simulink model "test_model_new1"  (R2018a)
settings: Solver=VariableStepAuto  StartTime=0.0  StopTime=7.1  RelTol=1e-3
values from neighbouring files (symbols this model uses):
  A = sys_d.A    [discreteTest.m]    (also in discreteTestAttacked.m)
  B = sys_d.B    [discreteTest.m]    (also in discreteTestAttacked.m)
  C = sys_d.C    [discreteTest.m]    (also in discreteTestAttacked.m)
  K = [   5.261, -0.023 ... (first row only)    [discreteTest.m]    (also in discreteTestAttacked.m)
  steeringAngle = zeros(1, time)    [discreteTest.m]    (also in discreteTestAttacked.m)
  Ts = 0.04    [discreteTest.m]    (also in discreteTestAttacked.m)
undefined symbols (not defined in the file or in its folder): canChannel, L
libraries: canlib x10, canmsglib x8, simulink x6
settings Model: Creator=Shreyash  LastModifiedBy=Shreyash

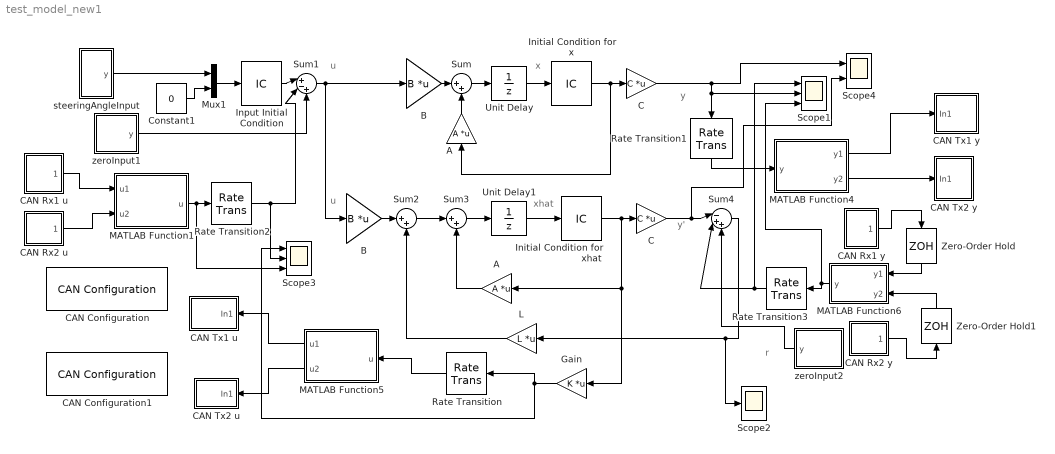
== system test_model_new1 ==
  note: y
  note: r
  note: y'
  note: u
  note: u
  note: x
  note: xhat
  A : Gain  Gain=A  Multiplication=Matrix(K*u)
  "A " : Gain  Gain=A  Multiplication=Matrix(K*u)
  B : Gain  Gain=B  Multiplication=Matrix(K*u)
  "B " : Gain  Gain=B  Multiplication=Matrix(K*u)
  C : Gain  Gain=C  Multiplication=Matrix(K*u)
  "C " : Gain  Gain=C  Multiplication=Matrix(K*u)
  CAN Configuration : canlib/CAN Configuration  BlockHandle=1047.0007  DeviceMenu=MathWorks Virtual 1 (Channel 1)  Device=MathWorks Virtual 1 (Channel 1)  ObjConstructor=canChannel('MathWorks', 'Virtual 1', 1)  BusSpeed=500000  EnableBitParameters=off  AckMode=Normal
      settings: SourceProductBaseCode=VN
  CAN Configuration1 : canlib/CAN Configuration  BlockHandle=1049.0009  DeviceMenu=MathWorks Virtual 1 (Channel 2)  Device=MathWorks Virtual 1 (Channel 2)  ObjConstructor=canChannel('MathWorks', 'Virtual 1', 2)  BusSpeed=500000  EnableBitParameters=off  AckMode=Normal
      settings: SourceProductBaseCode=VN
  CAN Rx1 u : Subsystem
  CAN Rx1 y : Subsystem
  CAN Rx2 u : Subsystem
  CAN Rx2 y : Subsystem
  CAN Tx1 u : Subsystem
  CAN Tx1 y : Subsystem
  CAN Tx2 u : Subsystem
  CAN Tx2 y : Subsystem
  Constant1 : Constant  Value=0
  Gain : Gain  Gain=K  Multiplication=Matrix(K*u)
  Initial Condition for x : InitialCondition  Value=[0;0]
  Initial Condition for xhat : InitialCondition  Value=[0;0]
  Input Initial Condition : InitialCondition  Value=[0;0]
  L : Gain  Gain=L  Multiplication=Matrix(K*u)
  MATLAB Function1 : MATLAB Function  TreatAsAtomicUnit=on
  MATLAB Function4 : MATLAB Function  TreatAsAtomicUnit=on
  MATLAB Function5 : MATLAB Function  TreatAsAtomicUnit=on
  MATLAB Function6 : MATLAB Function  TreatAsAtomicUnit=on
  Mux1 : Mux  Inputs=2
  Rate Transition : RateTransition  Deterministic=off  InitialCondition=Ts/500  OutPortSampleTime=Ts/500
  Rate Transition1 : RateTransition  Deterministic=off  InitialCondition=Ts  OutPortSampleTime=Ts
  Rate Transition2 : RateTransition  Deterministic=off  InitialCondition=0.0004  OutPortSampleTime=Ts
  Rate Transition3 : RateTransition  Deterministic=off  InitialCondition=0.0004  OutPortSampleTime=Ts/2
  Scope1 : Scope  NumInputPorts=3
  Scope2 : Scope
  Scope3 : Scope  NumInputPorts=3
  Scope4 : Scope  NumInputPorts=2
  Sum : Sum  Inputs=|++
  Sum1 : Sum  Inputs=|+-+
  Sum2 : Sum  Inputs=|++
  Sum3 : Sum  Inputs=|++
  Sum4 : Sum  Inputs=|-++
  Unit Delay : UnitDelay  SampleTime=-1
  Unit Delay1 : UnitDelay  SampleTime=-1
  Zero-Order Hold : ZeroOrderHold  SampleTime=Ts/100
  Zero-Order Hold1 : ZeroOrderHold  SampleTime=Ts/100
  steeringAngleInput : Subsystem
  zeroInput1 : Subsystem
  zeroInput2 : Subsystem
  wires:
  "B "/1 -> Sum/1
  Unit Delay/1 -> Initial Condition for x/1
  Sum/1 -> Unit Delay/1
  "A "/1 -> Sum/2
  Constant1/1 -> Mux1/2
  B/1 -> Sum2/1
  Sum2/1 -> Sum3/1
  Sum3/1 -> Unit Delay1/1
  Unit Delay1/1 -> Initial Condition for xhat/1
  L/1 -> Sum2/2
  A/1 -> Sum3/2
  Initial Condition for x/1 -> "C "/1, "A "/1
  C/1 -> Scope4/2, Sum4/1
  Initial Condition for xhat/1 -> C/1, A/1, Gain/1
  Mux1/1 -> Input Initial Condition/1
  Input Initial Condition/1 -> Sum1/1
  Gain/1 -> Scope3/1, Rate Transition/1
  Rate Transition/1 -> MATLAB Function5/1(u)
  "C "/1 -> Rate Transition1/1, Scope1/2, Scope4/1
  MATLAB Function5/1(u1) -> CAN Tx1 u/1(In1)
  MATLAB Function5/2(u2) -> CAN Tx2 u/1(In1)
  steeringAngleInput/1(y) -> Mux1/1
  zeroInput1/1(y) -> Sum1/3
  zeroInput2/1(y) -> Sum4/3
  CAN Rx2 u/1(Data) -> MATLAB Function1/2(u2)
  CAN Rx1 u/1(Data) -> MATLAB Function1/1(u1)
  MATLAB Function1/1(u) -> Scope3/3, Rate Transition2/1
  Sum1/1 -> "B "/1, B/1
  Sum4/1 -> Scope2/1, L/1
  Rate Transition2/1 -> Sum1/2, Scope3/2
  MATLAB Function6/1(y) -> Rate Transition3/1, Scope1/3
  Rate Transition3/1 -> Scope1/1, Sum4/2
  MATLAB Function4/1(y1) -> CAN Tx1 y/1(In1)
  MATLAB Function4/2(y2) -> CAN Tx2 y/1(In1)
  CAN Rx1 y/1(Data) -> Zero-Order Hold/1
  Zero-Order Hold/1 -> MATLAB Function6/1(y1)
  CAN Rx2 y/1(Data) -> Zero-Order Hold1/1
  Zero-Order Hold1/1 -> MATLAB Function6/2(y2)
  Rate Transition1/1 -> MATLAB Function4/1(y)

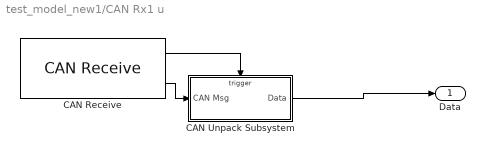
== system test_model_new1/CAN Rx1 u ==
  CAN Receive : canlib/CAN Receive  BlockHandle=1067.0006  DeviceMenu=MathWorks Virtual 1 (Channel 2)  Device=MathWorks Virtual 1 (Channel 2)  ObjConstructor=canChannel('MathWorks', 'Virtual 1', 2)  EnableStandardIDsFilter=off  StandardIDs=201  EnableExtendedIDsFilter=off  ExtendedIDs=0  SampleTime=0.0004  MsgsPerTimestep=all  StdIDsCombo=Allow only  ExtIDsCombo=Block all  InternalFilterUpdateStatus=on  BusOutput=off
      settings: SourceProductBaseCode=VN
  CAN Unpack Subsystem : Subsystem  TreatAsAtomicUnit=on
  Data : Outport  VectorParamsAs1DForOutWhenUnconnected=on
  wires:
  CAN Receive/2 -> CAN Unpack Subsystem/1(CAN Msg)
  CAN Receive/1 -> CAN Unpack Subsystem/Trigger
  CAN Unpack Subsystem/1(Data) -> Data/1

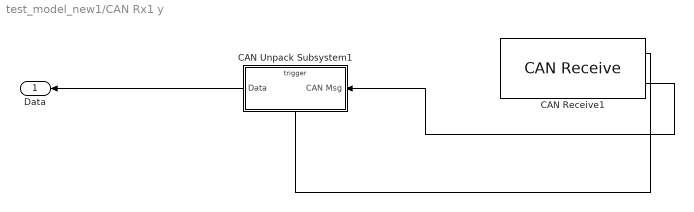
== system test_model_new1/CAN Rx1 y ==
  CAN Receive1 : canlib/CAN Receive  BlockHandle=1080.0006  DeviceMenu=MathWorks Virtual 1 (Channel 2)  Device=MathWorks Virtual 1 (Channel 2)  ObjConstructor=canChannel('MathWorks', 'Virtual 1', 2)  EnableStandardIDsFilter=off  StandardIDs=100  EnableExtendedIDsFilter=off  ExtendedIDs=0  SampleTime=0.0004  MsgsPerTimestep=all  StdIDsCombo=Allow only  ExtIDsCombo=Block all  InternalFilterUpdateStatus=on  BusOutput=off
      settings: SourceProductBaseCode=VN
  CAN Unpack Subsystem1 : Subsystem  TreatAsAtomicUnit=on
  Data : Outport  SampleTime=Ts  VectorParamsAs1DForOutWhenUnconnected=on
  wires:
  CAN Receive1/1 -> CAN Unpack Subsystem1/Trigger
  CAN Receive1/2 -> CAN Unpack Subsystem1/1(CAN Msg)
  CAN Unpack Subsystem1/1(Data) -> Data/1

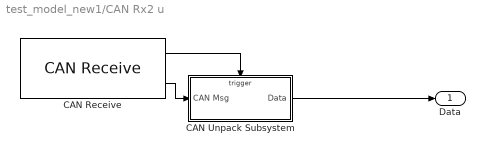
== system test_model_new1/CAN Rx2 u ==
  CAN Receive : canlib/CAN Receive  BlockHandle=1093.0005  DeviceMenu=MathWorks Virtual 1 (Channel 2)  Device=MathWorks Virtual 1 (Channel 2)  ObjConstructor=canChannel('MathWorks', 'Virtual 1', 2)  EnableStandardIDsFilter=off  StandardIDs=202  EnableExtendedIDsFilter=off  ExtendedIDs=0  SampleTime=0.0004  MsgsPerTimestep=all  StdIDsCombo=Allow only  ExtIDsCombo=Block all  InternalFilterUpdateStatus=on  BusOutput=off
      settings: SourceProductBaseCode=VN
  CAN Unpack Subsystem : Subsystem  TreatAsAtomicUnit=on
  Data : Outport  VectorParamsAs1DForOutWhenUnconnected=on
  wires:
  CAN Receive/2 -> CAN Unpack Subsystem/1(CAN Msg)
  CAN Receive/1 -> CAN Unpack Subsystem/Trigger
  CAN Unpack Subsystem/1(Data) -> Data/1

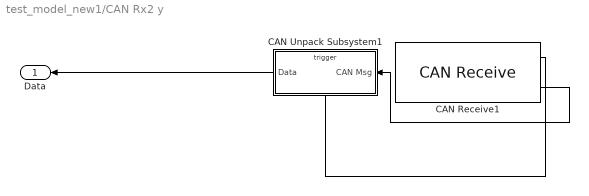
== system test_model_new1/CAN Rx2 y ==
  CAN Receive1 : canlib/CAN Receive  BlockHandle=1201.0005  DeviceMenu=MathWorks Virtual 1 (Channel 2)  Device=MathWorks Virtual 1 (Channel 2)  ObjConstructor=canChannel('MathWorks', 'Virtual 1', 2)  EnableStandardIDsFilter=off  StandardIDs=101  EnableExtendedIDsFilter=off  ExtendedIDs=0  SampleTime=0.0004  MsgsPerTimestep=all  StdIDsCombo=Allow only  ExtIDsCombo=Block all  InternalFilterUpdateStatus=on  BusOutput=off
      settings: SourceProductBaseCode=VN
  CAN Unpack Subsystem1 : Subsystem  TreatAsAtomicUnit=on
  Data : Outport  SampleTime=Ts  VectorParamsAs1DForOutWhenUnconnected=on
  wires:
  CAN Receive1/1 -> CAN Unpack Subsystem1/Trigger
  CAN Receive1/2 -> CAN Unpack Subsystem1/1(CAN Msg)
  CAN Unpack Subsystem1/1(Data) -> Data/1

== system test_model_new1/CAN Tx1 u ==
  In1 : Inport
  CAN Pack : canmsglib/CAN Pack  MsgList=(none)  MsgName=CAN Msg  MsgIDType=Standard (11-bit identifier)  MsgIdentifier=201  MsgLength=8  SignalInfo=signal$0$64$1$4$1$0$1$0$-Inf$Inf$#  NSignals=1  StartBits=str2num('[int32(0)]')  SignalSizes=str2num('[int32(64)]')  ByteOrders=str2num('[int32(1)]')  DataTypes=str2num('[int32(4)]')  MultiplexTypes=str2num('[int32(1)]')  MultiplexValues=str2num('[double(0)]')  Factors=str2num('[double(1)]')  Offsets=str2num('[double(0)]')  Minimums=str2num('[double(-Inf)]')  Maximums=str2num('[double(Inf)]')  Remote=off  ApplyMinMax=off  BusOutput=off
      settings: SourceProductBaseCode=ME,VN  DataFormat=manually specified signals
  CAN Transmit : canlib/CAN Transmit  BlockHandle=1258.0005  DeviceMenu=MathWorks Virtual 1 (Channel 1)  Device=MathWorks Virtual 1 (Channel 1)  ObjConstructor=canChannel('MathWorks', 'Virtual 1', 1)  EnablePeriodicTransmit=off  MessagePeriod=0.04
      settings: SourceProductBaseCode=VN
  wires:
  CAN Pack/1 -> CAN Transmit/1
  In1/1 -> CAN Pack/1

== system test_model_new1/CAN Tx1 y ==
  In1 : Inport
  CAN Pack1 : canmsglib/CAN Pack  MsgList=(none)  MsgName=CAN Msg  MsgIDType=Standard (11-bit identifier)  MsgIdentifier=100  MsgLength=8  SignalInfo=signal$0$64$1$4$1$0$1$0$-Inf$Inf$#  NSignals=1  StartBits=str2num('[int32(0)]')  SignalSizes=str2num('[int32(64)]')  ByteOrders=str2num('[int32(1)]')  DataTypes=str2num('[int32(4)]')  MultiplexTypes=str2num('[int32(1)]')  MultiplexValues=str2num('[double(0)]')  Factors=str2num('[double(1)]')  Offsets=str2num('[double(0)]')  Minimums=str2num('[double(-Inf)]')  Maximums=str2num('[double(Inf)]')  Remote=off  ApplyMinMax=off  BusOutput=off
      settings: SourceProductBaseCode=ME,VN  DataFormat=manually specified signals
  CAN Transmit1 : canlib/CAN Transmit  BlockHandle=1264.0005  DeviceMenu=MathWorks Virtual 1 (Channel 1)  Device=MathWorks Virtual 1 (Channel 1)  ObjConstructor=canChannel('MathWorks', 'Virtual 1', 1)  EnablePeriodicTransmit=off  MessagePeriod=0.04
      settings: SourceProductBaseCode=VN
  wires:
  In1/1 -> CAN Pack1/1
  CAN Pack1/1 -> CAN Transmit1/1

== system test_model_new1/CAN Tx2 u ==
  In1 : Inport
  CAN Pack : canmsglib/CAN Pack  MsgList=(none)  MsgName=CAN Msg  MsgIDType=Standard (11-bit identifier)  MsgIdentifier=202  MsgLength=8  SignalInfo=signal$0$64$1$4$1$0$1$0$-Inf$Inf$#  NSignals=1  StartBits=str2num('[int32(0)]')  SignalSizes=str2num('[int32(64)]')  ByteOrders=str2num('[int32(1)]')  DataTypes=str2num('[int32(4)]')  MultiplexTypes=str2num('[int32(1)]')  MultiplexValues=str2num('[double(0)]')  Factors=str2num('[double(1)]')  Offsets=str2num('[double(0)]')  Minimums=str2num('[double(-Inf)]')  Maximums=str2num('[double(Inf)]')  Remote=off  ApplyMinMax=off  BusOutput=off
      settings: SourceProductBaseCode=ME,VN  DataFormat=manually specified signals
  CAN Transmit : canlib/CAN Transmit  BlockHandle=1270.0005  DeviceMenu=MathWorks Virtual 1 (Channel 1)  Device=MathWorks Virtual 1 (Channel 1)  ObjConstructor=canChannel('MathWorks', 'Virtual 1', 1)  EnablePeriodicTransmit=off  MessagePeriod=0.04
      settings: SourceProductBaseCode=VN
  wires:
  CAN Pack/1 -> CAN Transmit/1
  In1/1 -> CAN Pack/1

== system test_model_new1/CAN Tx2 y ==
  In1 : Inport
  CAN Pack1 : canmsglib/CAN Pack  MsgList=(none)  MsgName=CAN Msg  MsgIDType=Standard (11-bit identifier)  MsgIdentifier=101  MsgLength=8  SignalInfo=signal$0$64$1$4$1$0$1$0$-Inf$Inf$#  NSignals=1  StartBits=str2num('[int32(0)]')  SignalSizes=str2num('[int32(64)]')  ByteOrders=str2num('[int32(1)]')  DataTypes=str2num('[int32(4)]')  MultiplexTypes=str2num('[int32(1)]')  MultiplexValues=str2num('[double(0)]')  Factors=str2num('[double(1)]')  Offsets=str2num('[double(0)]')  Minimums=str2num('[double(-Inf)]')  Maximums=str2num('[double(Inf)]')  Remote=off  ApplyMinMax=off  BusOutput=off
      settings: SourceProductBaseCode=ME,VN  DataFormat=manually specified signals
  CAN Transmit1 : canlib/CAN Transmit  BlockHandle=1276.0005  DeviceMenu=MathWorks Virtual 1 (Channel 1)  Device=MathWorks Virtual 1 (Channel 1)  ObjConstructor=canChannel('MathWorks', 'Virtual 1', 1)  EnablePeriodicTransmit=off  MessagePeriod=0.04
      settings: SourceProductBaseCode=VN
  wires:
  In1/1 -> CAN Pack1/1
  CAN Pack1/1 -> CAN Transmit1/1

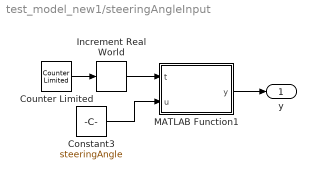
== system test_model_new1/steeringAngleInput ==
  Constant3 : Constant  Value=steeringAngle  SampleTime=Ts
  Counter Limited : simulink/Sources/Counter Limited  uplimit=size(steeringAngle,2)-1  tsamp=Ts
  Increment Real World : simulink/Additional Math & Discrete/Additional Math: Increment - Decrement/Increment Real World
      settings: SourceProductBaseCode=SL
  MATLAB Function1 : MATLAB Function  TreatAsAtomicUnit=on
  y : Outport  VectorParamsAs1DForOutWhenUnconnected=on
  wires:
  Counter Limited/1 -> Increment Real World/1
  Increment Real World/1 -> MATLAB Function1/1(t)
  MATLAB Function1/1(y) -> y/1
  Constant3/1 -> MATLAB Function1/2(u)

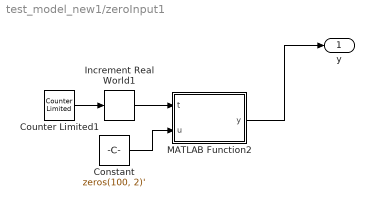
== system test_model_new1/zeroInput1 ==
  Constant : Constant  Value=zeros(100, 2)'
  Counter Limited1 : simulink/Sources/Counter Limited  uplimit=99  tsamp=0.04
  Increment Real World1 : simulink/Additional Math & Discrete/Additional Math: Increment - Decrement/Increment Real World
      settings: SourceProductBaseCode=SL
  MATLAB Function2 : MATLAB Function  TreatAsAtomicUnit=on
  y : Outport  VectorParamsAs1DForOutWhenUnconnected=on
  wires:
  Increment Real World1/1 -> MATLAB Function2/1(t)
  Counter Limited1/1 -> Increment Real World1/1
  Constant/1 -> MATLAB Function2/2(u)
  MATLAB Function2/1(y) -> y/1

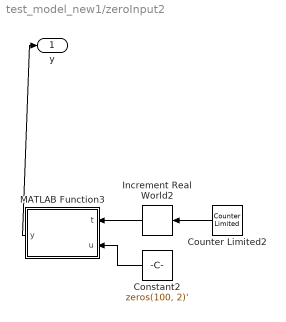
== system test_model_new1/zeroInput2 ==
  Constant2 : Constant  Value=zeros(100, 2)'
  Counter Limited2 : simulink/Sources/Counter Limited  uplimit=99  tsamp=0.04
  Increment Real World2 : simulink/Additional Math & Discrete/Additional Math: Increment - Decrement/Increment Real World
      settings: SourceProductBaseCode=SL
  MATLAB Function3 : MATLAB Function  TreatAsAtomicUnit=on
  y : Outport  VectorParamsAs1DForOutWhenUnconnected=on
  wires:
  Increment Real World2/1 -> MATLAB Function3/1(t)
  Counter Limited2/1 -> Increment Real World2/1
  Constant2/1 -> MATLAB Function3/2(u)
  MATLAB Function3/1(y) -> y/1

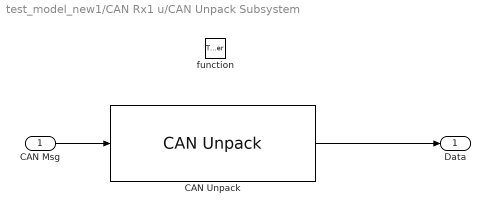
== system test_model_new1/CAN Rx1 u/CAN Unpack Subsystem ==
  CAN Msg : Inport
  function : TriggerPort  TriggerType=function-call  VariantControl=Variant
  CAN Unpack : canmsglib/CAN Unpack  MsgList=(none)  MsgName=CAN Msg  MsgIDType=Standard (11-bit identifier)  MsgIdentifier=201  MsgLength=8  SignalInfo=signal1$0$64$1$4$1$0$1$0$-Inf$Inf$#  NSignals=1  IDPort=off  TimestampPort=off  ErrorPort=off  RemotePort=off  LengthPort=off  StatusPort=off  StartBits=str2num('[int32(0)]')  SignalSizes=str2num('[int32(64)]')  ByteOrders=str2num('[int32(1)]')  DataTypes=str2num('[int32(4)]')  MultiplexTypes=str2num('[int32(1)]')  MultiplexValues=str2num('[double(0)]')  Factors=str2num('[double(1)]')  Offsets=str2num('[double(0)]')  Minimums=str2num('[double(-Inf)]')  Maximums=str2num('[double(Inf)]')  ApplyMinMax=off
      settings: SourceProductBaseCode=ME,VN
  Data : Outport
  wires:
  CAN Msg/1 -> CAN Unpack/1
  CAN Unpack/1 -> Data/1

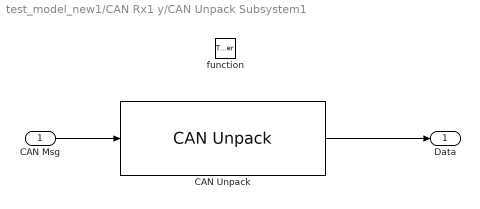
== system test_model_new1/CAN Rx1 y/CAN Unpack Subsystem1 ==
  CAN Msg : Inport
  function : TriggerPort  TriggerType=function-call  VariantControl=Variant
  CAN Unpack : canmsglib/CAN Unpack  MsgList=(none)  MsgName=CAN Msg  MsgIDType=Standard (11-bit identifier)  MsgIdentifier=100  MsgLength=8  SignalInfo=Signal1$0$64$1$4$1$0$1$0$-Inf$Inf$#  NSignals=1  IDPort=off  TimestampPort=off  ErrorPort=off  RemotePort=off  LengthPort=off  StatusPort=off  StartBits=str2num('[int32(0)]')  SignalSizes=str2num('[int32(64)]')  ByteOrders=str2num('[int32(1)]')  DataTypes=str2num('[int32(4)]')  MultiplexTypes=str2num('[int32(1)]')  MultiplexValues=str2num('[double(0)]')  Factors=str2num('[double(1)]')  Offsets=str2num('[double(0)]')  Minimums=str2num('[double(-Inf)]')  Maximums=str2num('[double(Inf)]')  ApplyMinMax=off
      settings: SourceProductBaseCode=ME,VN
  Data : Outport  OutputWhenDisabled=reset  InitialOutput=[0]
  wires:
  CAN Msg/1 -> CAN Unpack/1
  CAN Unpack/1 -> Data/1

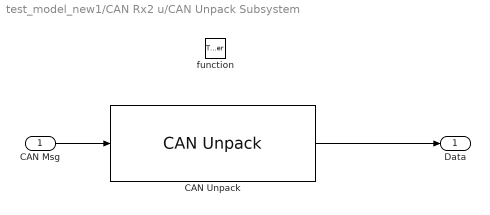
== system test_model_new1/CAN Rx2 u/CAN Unpack Subsystem ==
  CAN Msg : Inport
  function : TriggerPort  TriggerType=function-call  VariantControl=Variant
  CAN Unpack : canmsglib/CAN Unpack  MsgList=(none)  MsgName=CAN Msg  MsgIDType=Standard (11-bit identifier)  MsgIdentifier=202  MsgLength=8  SignalInfo=signal1$0$64$1$4$1$0$1$0$-Inf$Inf$#  NSignals=1  IDPort=off  TimestampPort=off  ErrorPort=off  RemotePort=off  LengthPort=off  StatusPort=off  StartBits=str2num('[int32(0)]')  SignalSizes=str2num('[int32(64)]')  ByteOrders=str2num('[int32(1)]')  DataTypes=str2num('[int32(4)]')  MultiplexTypes=str2num('[int32(1)]')  MultiplexValues=str2num('[double(0)]')  Factors=str2num('[double(1)]')  Offsets=str2num('[double(0)]')  Minimums=str2num('[double(-Inf)]')  Maximums=str2num('[double(Inf)]')  ApplyMinMax=off
      settings: SourceProductBaseCode=ME,VN
  Data : Outport
  wires:
  CAN Msg/1 -> CAN Unpack/1
  CAN Unpack/1 -> Data/1

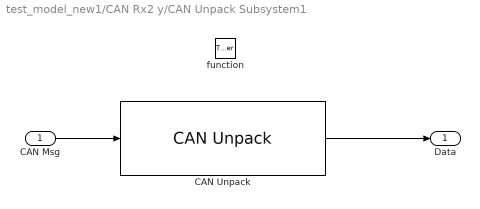
== system test_model_new1/CAN Rx2 y/CAN Unpack Subsystem1 ==
  CAN Msg : Inport
  function : TriggerPort  TriggerType=function-call  VariantControl=Variant
  CAN Unpack : canmsglib/CAN Unpack  MsgList=(none)  MsgName=CAN Msg  MsgIDType=Standard (11-bit identifier)  MsgIdentifier=101  MsgLength=8  SignalInfo=Signal1$0$64$1$4$1$0$1$0$-Inf$Inf$#  NSignals=1  IDPort=off  TimestampPort=off  ErrorPort=off  RemotePort=off  LengthPort=off  StatusPort=off  StartBits=str2num('[int32(0)]')  SignalSizes=str2num('[int32(64)]')  ByteOrders=str2num('[int32(1)]')  DataTypes=str2num('[int32(4)]')  MultiplexTypes=str2num('[int32(1)]')  MultiplexValues=str2num('[double(0)]')  Factors=str2num('[double(1)]')  Offsets=str2num('[double(0)]')  Minimums=str2num('[double(-Inf)]')  Maximums=str2num('[double(Inf)]')  ApplyMinMax=off
      settings: SourceProductBaseCode=ME,VN
  Data : Outport  OutputWhenDisabled=reset  InitialOutput=[0]
  wires:
  CAN Msg/1 -> CAN Unpack/1
  CAN Unpack/1 -> Data/1

== matlab function test_model_new1/steeringAngleInput/MATLAB Function1 ==
  data: t input; u input; y output
function y = fcn(t, u)
y = u(t)*(pi/180)*0.0625;
%for t = 1 :100
    %y = au(:, t);
    %y = (-1 + 2.*rand(1, 2))'; 
end

== matlab function test_model_new1/zeroInput1/MATLAB Function2 ==
  data: t input; u input; y output
function y = fcn(t, u)
y = u(:, t);
%for t = 1 :100
    %y = au(:, t);
    %y = (-1 + 2.*rand(1, 2))'; 
end

== matlab function test_model_new1/zeroInput2/MATLAB Function3 ==
  data: t input; u input; y output
function y = fcn(t, u)
y = u(:, t);
%for t = 1 :100
    %y = au(:, t);
    %y = (-1 + 2.*rand(1, 2))'; 
end

== matlab function test_model_new1/MATLAB Function4 ==
  data: y input; y1 output; y2 output
function [y1,y2] = fcn(y)
y1=y(1,1);
y2=y(2,1);
end

== matlab function test_model_new1/MATLAB Function5 ==
  data: u input; u1 output; u2 output
function [u1,u2] = fcn(u)
u1=u(1,1);
u2=u(2,1);
end

== matlab function test_model_new1/MATLAB Function6 ==
  data: y1 input; y output; y2 input
function y = fcn(y1,y2)
y=[y1;y2];
end

== matlab function test_model_new1/MATLAB Function1 ==
  data: u1 input; u output; u2 input
function u = fcn(u1,u2)
u=[u1;u2];
end
